simulink model "robot_soccer_sim_old"  (R2013a)
settings: Solver=ode45  StartTime=0.0  StopTime=1000000  RelTol=1e-3
InitFcn:
  | param
undefined symbols (not defined in the file or in its folder): controller_away_full_state, controller_home_full_state, drawEnvironment_est, lowlevelctrl, observer, P, robot_change_frames, vision_system
settings Model: Creator=beard  LastModifiedBy=beard

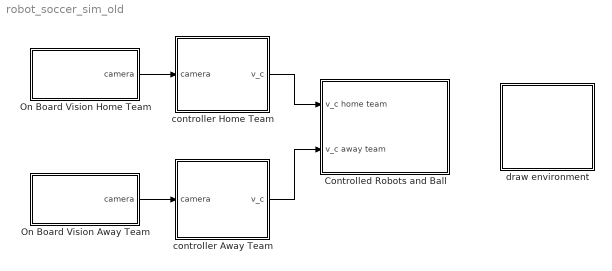
== system robot_soccer_sim_old ==
  "Controlled Robots and Ball " : Subsystem
      mask Display: image(imread('cmu_2002_diffbot.jpg'))
  On Board Vision Away Team : Subsystem
      mask Display: image(imread('softkinect.png'))
  On Board Vision Home Team : Subsystem
      mask Display: image(imread('softkinect.png'))
  controller Away Team : Subsystem
      mask Display: image(imread('minnowboard.png'))
  controller Home Team : Subsystem
      mask Display: image(imread('minnowboard.png'))
  draw environment : Subsystem
      mask Display: image(imread('ssl_game.jpg'))
  wires:
  controller Away Team/1(v_c) -> "Controlled Robots and Ball "/2(v_c away team)
  controller Home Team/1(v_c) -> "Controlled Robots and Ball "/1(v_c home team)
  On Board Vision Home Team/1(camera) -> controller Home Team/1(camera)
  On Board Vision Away Team/1(camera) -> controller Away Team/1(camera)

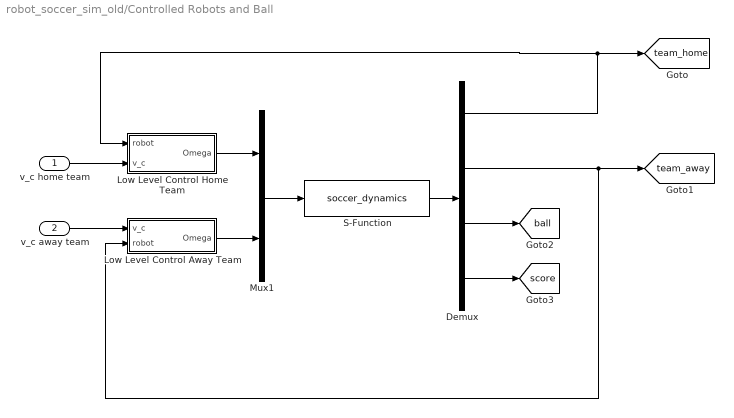
== system robot_soccer_sim_old/Controlled Robots and Ball  ==
  v_c home team : Inport
  v_c away team : Inport  Port=2
  Demux : Demux  Outputs=[3*P.num_robots; 3*P.num_robots; 2; 2]
  Low Level Control Home Team : Subsystem
  Low Level Control Away Team : Subsystem
  Mux1 : Mux  Inputs=2
  S-Function : S-Function  FunctionName=soccer_dynamics  Parameters=P  EnableBusSupport=off
  tag scope: ball=global, score=global, team_away=global, team_home=global
  wires:
  Demux/4 -> [score]
  v_c away team/1 -> Low Level Control Away Team/1(v_c)
  v_c home team/1 -> Low Level Control Home Team/2(v_c)
  Demux/2 -> [team_away], Low Level Control Away Team/2(robot)
  Low Level Control Away Team/1(Omega) -> Mux1/2
  Low Level Control Home Team/1(Omega) -> Mux1/1
  Demux/1 -> [team_home], Low Level Control Home Team/1(robot)
  S-Function/1 -> Demux/1
  Demux/3 -> [ball]
  Mux1/1 -> S-Function/1

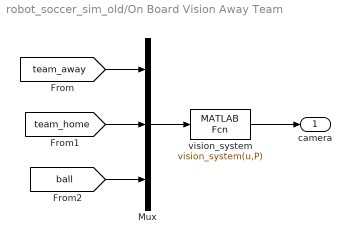
== system robot_soccer_sim_old/On Board Vision Away Team ==
  Mux : Mux  Inputs=3
  vision_system : MATLABFcn  MATLABFcn=vision_system(u,P)  OutputDimensions=(2+4*P.num_robots+2*P.num_markers)*P.num_robots  SampleTime=.01
  camera : Outport
  wires:
  Mux/1 -> vision_system/1
  [team_away] -> Mux/1
  [ball] -> Mux/3
  vision_system/1 -> camera/1
  [team_home] -> Mux/2

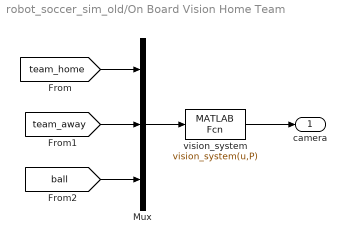
== system robot_soccer_sim_old/On Board Vision Home Team ==
  Mux : Mux  Inputs=3
  vision_system : MATLABFcn  MATLABFcn=vision_system(u,P)  OutputDimensions=(2+4*P.num_robots+2*P.num_markers)*P.num_robots  SampleTime=.01
  camera : Outport
  wires:
  Mux/1 -> vision_system/1
  [team_home] -> Mux/1
  [ball] -> Mux/3
  vision_system/1 -> camera/1
  [team_away] -> Mux/2

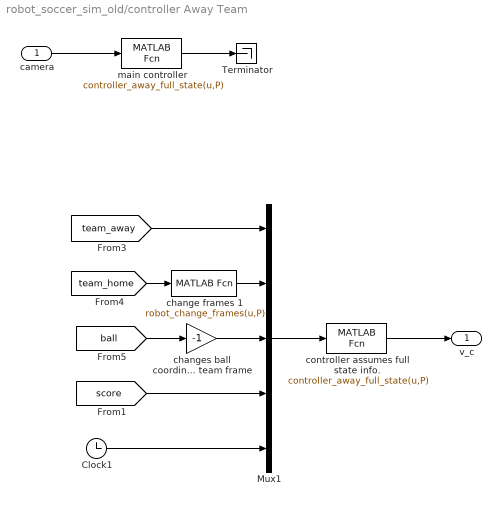
== system robot_soccer_sim_old/controller Away Team ==
  camera : Inport
  Clock1 : Clock
  Mux1 : Mux  Inputs=5
  Terminator : Terminator
  change frames 1 : MATLABFcn  MATLABFcn=robot_change_frames(u,P)  OutputDimensions=3*P.num_robots  SampleTime=P.control_sample_rate
  changes ball coordinates to away team frame : Gain  Gain=-1
  controller assumes full state info. : MATLABFcn  MATLABFcn=controller_away_full_state(u,P)  OutputDimensions=3*P.num_robots  SampleTime=P.control_sample_rate
  main controller : MATLABFcn  MATLABFcn=controller_away_full_state(u,P)  OutputDimensions=3*P.num_robots  SampleTime=0.01
  v_c : Outport
  wires:
  camera/1 -> main controller/1
  Mux1/1 -> controller assumes full state info./1
  [team_away] -> Mux1/1
  Clock1/1 -> Mux1/5
  controller assumes full state info./1 -> v_c/1
  change frames 1/1 -> Mux1/2
  [team_home] -> change frames 1/1
  [ball] -> changes ball coordinates to away team frame/1
  changes ball coordinates to away team frame/1 -> Mux1/3
  [score] -> Mux1/4
  main controller/1 -> Terminator/1

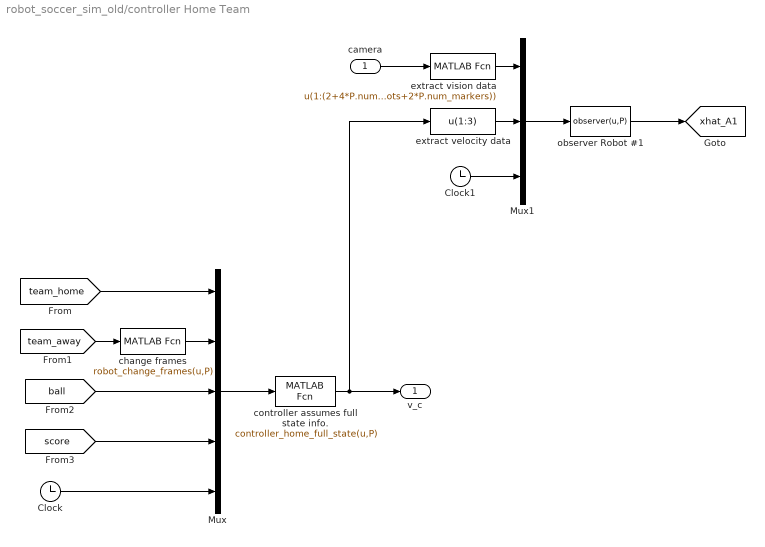
== system robot_soccer_sim_old/controller Home Team ==
  camera : Inport
  Clock : Clock
  Clock1 : Clock
  Mux : Mux  Inputs=5
  Mux1 : Mux  Inputs=3
  "change frames " : MATLABFcn  MATLABFcn=robot_change_frames(u,P)  OutputDimensions=3*P.num_robots  SampleTime=P.control_sample_rate
  controller assumes full state info. : MATLABFcn  MATLABFcn=controller_home_full_state(u,P)  OutputDimensions=3*P.num_robots  SampleTime=P.control_sample_rate
  extract velocity data : MATLABFcn  MATLABFcn=u(1:3)  OutputDimensions=3  SampleTime=P.control_sample_rate
  extract vision data : MATLABFcn  MATLABFcn=u(1:(2+4*P.num_robots+2*P.num_markers))  OutputDimensions=(2+4*P.num_robots+2*P.num_markers)  SampleTime=P.control_sample_rate
  observer Robot #1 : MATLABFcn  MATLABFcn=observer(u,P)  OutputDimensions=3+3*3  SampleTime=P.control_sample_rate
  v_c : Outport
  tag scope: xhat_A1=global
  wires:
  Mux/1 -> controller assumes full state info./1
  [team_home] -> Mux/1
  [ball] -> Mux/3
  Clock/1 -> Mux/5
  controller assumes full state info./1 -> extract velocity data/1, v_c/1
  camera/1 -> extract vision data/1
  Mux1/1 -> observer Robot #1/1
  extract vision data/1 -> Mux1/1
  Clock1/1 -> Mux1/3
  extract velocity data/1 -> Mux1/2
  observer Robot #1/1 -> [xhat_A1]
  "change frames "/1 -> Mux/2
  [team_away] -> "change frames "/1
  [score] -> Mux/4

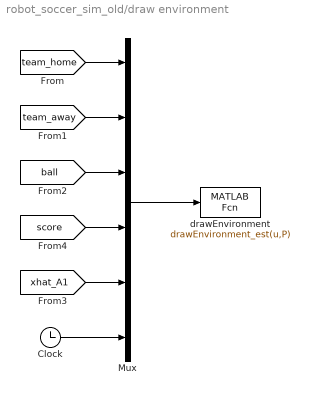
== system robot_soccer_sim_old/draw environment ==
  Clock : Clock
  Mux : Mux  Inputs=6
  drawEnvironment : MATLABFcn  MATLABFcn=drawEnvironment_est(u,P)  OutputDimensions=0  SampleTime=P.display_rate
  wires:
  Mux/1 -> drawEnvironment/1
  Clock/1 -> Mux/6
  [team_home] -> Mux/1
  [team_away] -> Mux/2
  [ball] -> Mux/3
  [xhat_A1] -> Mux/5
  [score] -> Mux/4

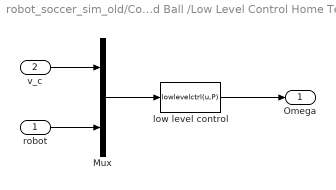
== system robot_soccer_sim_old/Controlled Robots and Ball /Low Level Control Home Team ==
  robot : Inport
  v_c : Inport  Port=2
  Mux : Mux  Inputs=2
  low level control : MATLABFcn  MATLABFcn=lowlevelctrl(u,P)  OutputDimensions=3*P.num_robots  SampleTime=0.01
  Omega : Outport
  wires:
  low level control/1 -> Omega/1
  Mux/1 -> low level control/1
  robot/1 -> Mux/2
  v_c/1 -> Mux/1

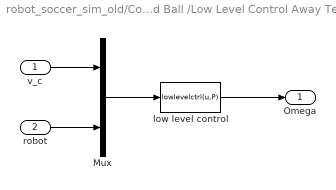
== system robot_soccer_sim_old/Controlled Robots and Ball /Low Level Control Away Team ==
  v_c : Inport
  robot : Inport  Port=2
  Mux : Mux  Inputs=2
  low level control : MATLABFcn  MATLABFcn=lowlevelctrl(u,P)  OutputDimensions=3*P.num_robots  SampleTime=0.01
  Omega : Outport
  wires:
  low level control/1 -> Omega/1
  Mux/1 -> low level control/1
  robot/1 -> Mux/2
  v_c/1 -> Mux/1
